simulink model "MyDriveLine_RTW"  (R2022a)
settings: Solver=ode1  StartTime=0.0  StopTime=inf  FixedStep=0.0002  RelTol=1e-3
PreLoadFcn:
  | vehicle = 'Car'; if ~length(which('cmcmd')), cmenv; end
  | MyDriveLine_RTW_bus
InitFcn:
  | vehicle = 'Car'; if ~length(which('cmcmd')), cmenv; end
  | MyDriveLine_RTW_bus
undefined symbols (not defined in the file or in its folder): DiscIntNeverNeededParam
libraries: simulink x3, CarMaker4SL x1
Description:
  | CarMaker Plug-in Model Target
settings Model: ModifiedByFormat=IPG  Creator=IPG  LastModifiedBy=IPG
settings SolverCC: AlgebraicLoopSolver=TrustRegion
settings DataIOCC: LimitDataPoints=on  SaveFormat=Array  SignalLoggingSaveFormat=ModelDataLogs  ReturnWorkspaceOutputs=off
settings OptimizationCC: ExpressionDepthLimit=2147483647  LifeSpan=inf
settings DebuggingCC: UnderspecifiedInitializationDetection=Classic  MergeDetectMultiDrivingBlocksExec=none  FcnCallInpInsideContextMsg=warning  UnconnectedInputMsg=warning  UnconnectedOutputMsg=warning  UnconnectedLineMsg=warning  StateNameClashWarn=warning  SFUnexpectedBacktrackingDiag=warning  SFNoUnconditionalDefaultTransitionDiag=warning  SFMachineParentedDataDiag=warning  ArithmeticOperatorsInVariantConditions=warning
settings HardwareCC: ProdBitPerPointer=32  ProdBitPerSizeT=32  ProdBitPerPtrDiffT=32  ProdLargestAtomicFloat=None  ProdIntDivRoundTo=Undefined  ProdEndianess=Unspecified  ProdWordSize=32  ProdHWDeviceType=32-bit Generic  TargetHWDeviceType=32-bit Generic  ProdEqTarget=off
settings ModelReferenceCC: PropagateSignalLabelsOutOfModel=off
settings SFSimCC: SimUseLocalCustomCode=off  CustomCodeUndefinedFunction=UseInterfaceOnly
settings RTWCC: Description=CarMaker Plug-in Model Target  SystemTargetFile=CarMaker.tlc  TemplateMakefile=CarMaker_unix-win64.tmf  RTWUseLocalCustomCode=off  CustomSourceCode="#include \"SimCore.h\""  DLArmComputeVersion=19.05
settings CodeAppCC: MaxIdLength=63  StateflowObjectComments=on
settings STFCustomTargetCC: ModelReferenceCompliant=off  CodeInterfacePackaging=Reusable function  CPPClassGenCompliant=on  GRTInterface=off  GenerateAllocFcn=on  SystemTargetFile=CarMaker.tlc
settings GRTTargetCC: TargetLangStandard=C89/C90 (ANSI)  ModelReferenceCompliant=off  ParMdlRefBuildCompliant=off  CompOptLevelCompliant=off  ConcurrentExecutionCompliant=off  CombineOutputUpdateFcns=off  MatFileLogging=off  CodeInterfacePackaging=Reusable function  GenerateAllocFcn=on  UseToolchainInfoCompliant=off  ExtModeMexFile=noextcomm
settings ConfigComp: CovMetricSettings=dw  CovSaveCumulativeToWorkspaceVar=on  CovSaveSingleToWorkspaceVar=on  CovExternalEMLEnable=off

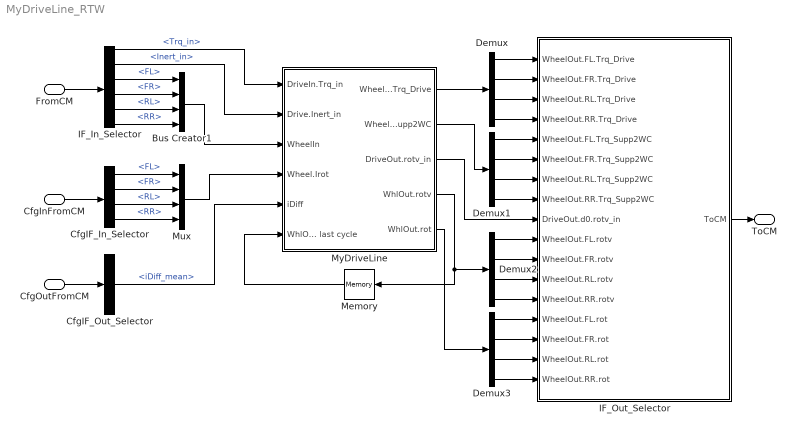
== system MyDriveLine_RTW ==
  FromCM : Inport  OutDataTypeStr=Bus: cmPTDriveLineIn
  CfgInFromCM : Inport  Port=2  OutDataTypeStr=Bus: cmPTDriveLineCfgIn
  CfgOutFromCM : Inport  Port=3  OutDataTypeStr=Bus: cmPTDriveLineCfgOut
  Bus Creator1 : BusCreator  Inputs=4
  CfgIF_In_Selector : BusSelector  OutputSignals=Wheel_Iyy.FL,Wheel_Iyy.FR,Wheel_Iyy.RL,Wheel_Iyy.RR
  CfgIF_Out_Selector : BusSelector  OutputSignals=iDiff_mean
  Demux{,1..3} (4 alike) : Demux
  IF_In_Selector : BusSelector  OutputSignals=DriveIn.d0.Trq_in,DriveIn.d0.Inert_in,WheelIn.FL,WheelIn.FR,WheelIn.RL,WheelIn.RR
  IF_Out_Selector : Subsystem  mask(Signal Selection){}
      mask help: Signal Selection Block
      settings: OpenFcn=cmSignalSelect('SignalSelection_CB',gcb)
  Memory : Memory
  Mux : Mux
  MyDriveLine : Subsystem
  ToCM : Outport  OutDataTypeStr=Bus: cmPTDriveLineOut  VectorParamsAs1DForOutWhenUnconnected=off
  wires:
  FromCM/1 -> IF_In_Selector/1
  IF_Out_Selector/1(ToCM) -> ToCM/1
  CfgInFromCM/1 -> CfgIF_In_Selector/1
  CfgOutFromCM/1 -> CfgIF_Out_Selector/1
  MyDriveLine/1(WheelOut.Trq_Drive) -> Demux/1
  CfgIF_Out_Selector/1 -> MyDriveLine/5(iDiff)  "<iDiff_mean>"
  Demux1/4 -> IF_Out_Selector/8(WheelOut.RR.Trq_Supp2WC)
  MyDriveLine/2(WheelOut.Trq_Supp2WC) -> Demux1/1
  Demux2/1 -> IF_Out_Selector/10(WheelOut.FL.rotv)
  Demux2/2 -> IF_Out_Selector/11(WheelOut.FR.rotv)
  Demux2/3 -> IF_Out_Selector/12(WheelOut.RL.rotv)
  Demux2/4 -> IF_Out_Selector/13(WheelOut.RR.rotv)
  MyDriveLine/4(WhlOut.rotv) -> Demux2/1, Memory/1
  Demux3/1 -> IF_Out_Selector/14(WheelOut.FL.rot)
  Demux3/2 -> IF_Out_Selector/15(WheelOut.FR.rot)
  Demux3/3 -> IF_Out_Selector/16(WheelOut.RL.rot)
  Demux3/4 -> IF_Out_Selector/17(WheelOut.RR.rot)
  MyDriveLine/5(WhlOut.rot) -> Demux3/1
  Memory/1 -> MyDriveLine/6(WhlOut.rotv last cycle)
  Mux/1 -> MyDriveLine/4(Wheel.Irot)
  Bus Creator1/1 -> MyDriveLine/3(WheelIn)
  Demux/1 -> IF_Out_Selector/1(WheelOut.FL.Trq_Drive)
  Demux/2 -> IF_Out_Selector/2(WheelOut.FR.Trq_Drive)
  Demux/3 -> IF_Out_Selector/3(WheelOut.RL.Trq_Drive)
  Demux/4 -> IF_Out_Selector/4(WheelOut.RR.Trq_Drive)
  Demux1/1 -> IF_Out_Selector/5(WheelOut.FL.Trq_Supp2WC)
  Demux1/2 -> IF_Out_Selector/6(WheelOut.FR.Trq_Supp2WC)
  Demux1/3 -> IF_Out_Selector/7(WheelOut.RL.Trq_Supp2WC)
  MyDriveLine/3(DriveOut.rotv_in) -> IF_Out_Selector/9(DriveOut.d0.rotv_in)
  CfgIF_In_Selector/1 -> Mux/1  "<FL>"
  CfgIF_In_Selector/2 -> Mux/2  "<FR>"
  CfgIF_In_Selector/3 -> Mux/3  "<RL>"
  CfgIF_In_Selector/4 -> Mux/4  "<RR>"
  IF_In_Selector/1 -> MyDriveLine/1(DriveIn.Trq_in)  "<Trq_in>"
  IF_In_Selector/2 -> MyDriveLine/2(Drive.Inert_in)  "<Inert_in>"
  IF_In_Selector/3 -> Bus Creator1/1  "<FL>"
  IF_In_Selector/4 -> Bus Creator1/2  "<FR>"
  IF_In_Selector/5 -> Bus Creator1/3  "<RL>"
  IF_In_Selector/6 -> Bus Creator1/4  "<RR>"

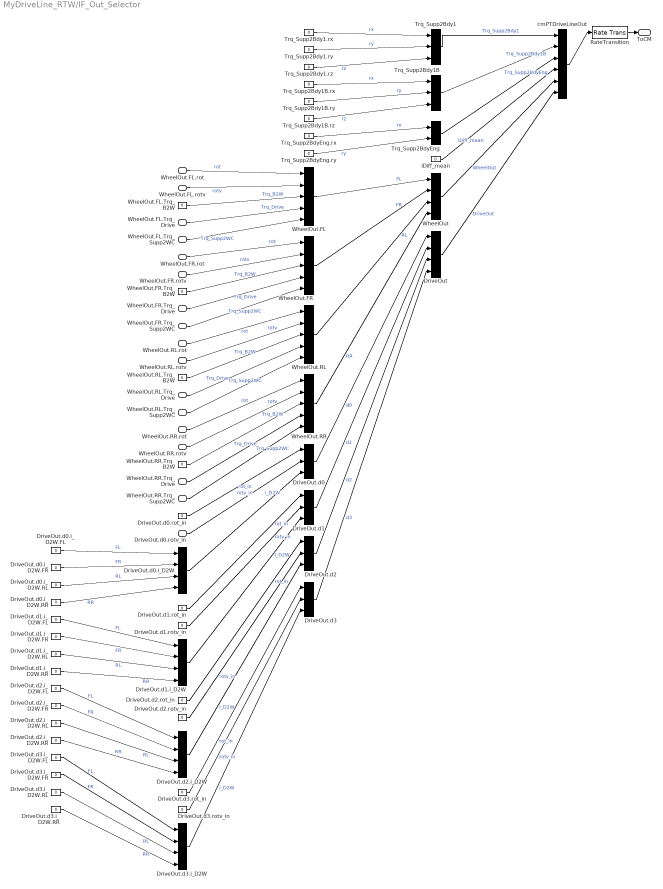
== system MyDriveLine_RTW/IF_Out_Selector ==
  WheelOut.FL.Trq_Drive : Inport
  WheelOut.FR.Trq_Drive : Inport  Port=2
  WheelOut.RL.Trq_Drive : Inport  Port=3
  WheelOut.RR.Trq_Drive : Inport  Port=4
  WheelOut.FL.Trq_Supp2WC : Inport  Port=5
  WheelOut.FR.Trq_Supp2WC : Inport  Port=6
  WheelOut.RL.Trq_Supp2WC : Inport  Port=7
  WheelOut.RR.Trq_Supp2WC : Inport  Port=8
  DriveOut.d0.rotv_in : Inport  Port=9
  WheelOut.FL.rotv : Inport  Port=10
  WheelOut.FR.rotv : Inport  Port=11
  WheelOut.RL.rotv : Inport  Port=12
  WheelOut.RR.rotv : Inport  Port=13
  WheelOut.FL.rot : Inport  Port=14
  WheelOut.FR.rot : Inport  Port=15
  WheelOut.RL.rot : Inport  Port=16
  WheelOut.RR.rot : Inport  Port=17
  DriveOut : BusCreator  Inputs=4
  DriveOut.d{0..3} (4 alike) : BusCreator  Inputs=3
  DriveOut.d0.i_D2W : BusCreator  Inputs=4
  DriveOut.d0.i_D2W.FL : Constant  Value=0
  DriveOut.d0.i_D2W.FR : Constant  Value=0
  DriveOut.d0.i_D2W.RL : Constant  Value=0
  DriveOut.d0.i_D2W.RR : Constant  Value=0
  DriveOut.d0.rot_in : Constant  Value=0
  DriveOut.d1.i_D2W : BusCreator  Inputs=4
  DriveOut.d1.i_D2W.FL : Constant  Value=0
  DriveOut.d1.i_D2W.FR : Constant  Value=0
  DriveOut.d1.i_D2W.RL : Constant  Value=0
  DriveOut.d1.i_D2W.RR : Constant  Value=0
  DriveOut.d1.rot_in : Constant  Value=0
  DriveOut.d1.rotv_in : Constant  Value=0
  DriveOut.d2.i_D2W : BusCreator  Inputs=4
  DriveOut.d2.i_D2W.FL : Constant  Value=0
  DriveOut.d2.i_D2W.FR : Constant  Value=0
  DriveOut.d2.i_D2W.RL : Constant  Value=0
  DriveOut.d2.i_D2W.RR : Constant  Value=0
  DriveOut.d2.rot_in : Constant  Value=0
  DriveOut.d2.rotv_in : Constant  Value=0
  DriveOut.d3.i_D2W : BusCreator  Inputs=4
  DriveOut.d3.i_D2W.FL : Constant  Value=0
  DriveOut.d3.i_D2W.FR : Constant  Value=0
  DriveOut.d3.i_D2W.RL : Constant  Value=0
  DriveOut.d3.i_D2W.RR : Constant  Value=0
  DriveOut.d3.rot_in : Constant  Value=0
  DriveOut.d3.rotv_in : Constant  Value=0
  RateTransition : RateTransition  OutPortSampleTime=str2num(get_param(bdroot,'FixedStep'))
  Trq_Supp2Bdy1 : BusCreator  Inputs=3
  Trq_Supp2Bdy1.rx : Constant  Value=0
  Trq_Supp2Bdy1.ry : Constant  Value=0
  Trq_Supp2Bdy1.rz : Constant  Value=0
  Trq_Supp2Bdy1B : BusCreator  Inputs=3
  Trq_Supp2Bdy1B.rx : Constant  Value=0
  Trq_Supp2Bdy1B.ry : Constant  Value=0
  Trq_Supp2Bdy1B.rz : Constant  Value=0
  Trq_Supp2BdyEng : BusCreator  Inputs=2
  Trq_Supp2BdyEng.rx : Constant  Value=0
  Trq_Supp2BdyEng.ry : Constant  Value=0
  WheelOut : BusCreator  Inputs=4
  WheelOut.FL : BusCreator  Inputs=5
  WheelOut.FL.Trq_B2W : Constant  Value=0
  WheelOut.FR : BusCreator  Inputs=5
  WheelOut.FR.Trq_B2W : Constant  Value=0
  WheelOut.RL : BusCreator  Inputs=5
  WheelOut.RL.Trq_B2W : Constant  Value=0
  WheelOut.RR : BusCreator  Inputs=5
  WheelOut.RR.Trq_B2W : Constant  Value=0
  cmPTDriveLineOut : BusCreator  Inputs=6
  iDiff_mean : Constant  Value=0
  ToCM : Outport  VectorParamsAs1DForOutWhenUnconnected=off
  wires:
  RateTransition/1 -> ToCM/1
  cmPTDriveLineOut/1 -> RateTransition/1
  Trq_Supp2Bdy1/1 -> cmPTDriveLineOut/1  "Trq_Supp2Bdy1"
  Trq_Supp2Bdy1.rx/1 -> Trq_Supp2Bdy1/1  "rx"
  Trq_Supp2Bdy1.ry/1 -> Trq_Supp2Bdy1/2  "ry"
  Trq_Supp2Bdy1.rz/1 -> Trq_Supp2Bdy1/3  "rz"
  Trq_Supp2Bdy1B/1 -> cmPTDriveLineOut/2  "Trq_Supp2Bdy1B"
  Trq_Supp2Bdy1B.rx/1 -> Trq_Supp2Bdy1B/1  "rx"
  Trq_Supp2Bdy1B.ry/1 -> Trq_Supp2Bdy1B/2  "ry"
  Trq_Supp2Bdy1B.rz/1 -> Trq_Supp2Bdy1B/3  "rz"
  Trq_Supp2BdyEng/1 -> cmPTDriveLineOut/3  "Trq_Supp2BdyEng"
  Trq_Supp2BdyEng.rx/1 -> Trq_Supp2BdyEng/1  "rx"
  Trq_Supp2BdyEng.ry/1 -> Trq_Supp2BdyEng/2  "ry"
  iDiff_mean/1 -> cmPTDriveLineOut/4  "iDiff_mean"
  WheelOut/1 -> cmPTDriveLineOut/5  "WheelOut"
  WheelOut.FL/1 -> WheelOut/1  "FL"
  WheelOut.FL.Trq_B2W/1 -> WheelOut.FL/3  "Trq_B2W"
  WheelOut.FR/1 -> WheelOut/2  "FR"
  WheelOut.FR.Trq_B2W/1 -> WheelOut.FR/3  "Trq_B2W"
  WheelOut.RL/1 -> WheelOut/3  "RL"
  WheelOut.RL.Trq_B2W/1 -> WheelOut.RL/3  "Trq_B2W"
  WheelOut.RR/1 -> WheelOut/4  "RR"
  WheelOut.RR.Trq_B2W/1 -> WheelOut.RR/3  "Trq_B2W"
  DriveOut/1 -> cmPTDriveLineOut/6  "DriveOut"
  DriveOut.d0/1 -> DriveOut/1  "d0"
  DriveOut.d0.rot_in/1 -> DriveOut.d0/1  "rot_in"
  DriveOut.d0.i_D2W/1 -> DriveOut.d0/3  "i_D2W"
  DriveOut.d0.i_D2W.FL/1 -> DriveOut.d0.i_D2W/1  "FL"
  DriveOut.d0.i_D2W.FR/1 -> DriveOut.d0.i_D2W/2  "FR"
  DriveOut.d0.i_D2W.RL/1 -> DriveOut.d0.i_D2W/3  "RL"
  DriveOut.d0.i_D2W.RR/1 -> DriveOut.d0.i_D2W/4  "RR"
  DriveOut.d1/1 -> DriveOut/2  "d1"
  DriveOut.d1.rot_in/1 -> DriveOut.d1/1  "rot_in"
  DriveOut.d1.rotv_in/1 -> DriveOut.d1/2  "rotv_in"
  DriveOut.d1.i_D2W/1 -> DriveOut.d1/3  "i_D2W"
  DriveOut.d1.i_D2W.FL/1 -> DriveOut.d1.i_D2W/1  "FL"
  DriveOut.d1.i_D2W.FR/1 -> DriveOut.d1.i_D2W/2  "FR"
  DriveOut.d1.i_D2W.RL/1 -> DriveOut.d1.i_D2W/3  "RL"
  DriveOut.d1.i_D2W.RR/1 -> DriveOut.d1.i_D2W/4  "RR"
  DriveOut.d2/1 -> DriveOut/3  "d2"
  DriveOut.d2.rot_in/1 -> DriveOut.d2/1  "rot_in"
  DriveOut.d2.rotv_in/1 -> DriveOut.d2/2  "rotv_in"
  DriveOut.d2.i_D2W/1 -> DriveOut.d2/3  "i_D2W"
  DriveOut.d2.i_D2W.FL/1 -> DriveOut.d2.i_D2W/1  "FL"
  DriveOut.d2.i_D2W.FR/1 -> DriveOut.d2.i_D2W/2  "FR"
  DriveOut.d2.i_D2W.RL/1 -> DriveOut.d2.i_D2W/3  "RL"
  DriveOut.d2.i_D2W.RR/1 -> DriveOut.d2.i_D2W/4  "RR"
  DriveOut.d3/1 -> DriveOut/4  "d3"
  DriveOut.d3.rot_in/1 -> DriveOut.d3/1  "rot_in"
  DriveOut.d3.rotv_in/1 -> DriveOut.d3/2  "rotv_in"
  DriveOut.d3.i_D2W/1 -> DriveOut.d3/3  "i_D2W"
  DriveOut.d3.i_D2W.FL/1 -> DriveOut.d3.i_D2W/1  "FL"
  DriveOut.d3.i_D2W.FR/1 -> DriveOut.d3.i_D2W/2  "FR"
  DriveOut.d3.i_D2W.RL/1 -> DriveOut.d3.i_D2W/3  "RL"
  DriveOut.d3.i_D2W.RR/1 -> DriveOut.d3.i_D2W/4  "RR"
  WheelOut.FL.Trq_Drive/1 -> WheelOut.FL/4  "Trq_Drive"
  WheelOut.FR.Trq_Drive/1 -> WheelOut.FR/4  "Trq_Drive"
  WheelOut.RL.Trq_Drive/1 -> WheelOut.RL/4  "Trq_Drive"
  WheelOut.RR.Trq_Drive/1 -> WheelOut.RR/4  "Trq_Drive"
  WheelOut.FL.Trq_Supp2WC/1 -> WheelOut.FL/5  "Trq_Supp2WC"
  WheelOut.FR.Trq_Supp2WC/1 -> WheelOut.FR/5  "Trq_Supp2WC"
  WheelOut.RL.Trq_Supp2WC/1 -> WheelOut.RL/5  "Trq_Supp2WC"
  WheelOut.RR.Trq_Supp2WC/1 -> WheelOut.RR/5  "Trq_Supp2WC"
  DriveOut.d0.rotv_in/1 -> DriveOut.d0/2  "rotv_in"
  WheelOut.FL.rotv/1 -> WheelOut.FL/2  "rotv"
  WheelOut.FR.rotv/1 -> WheelOut.FR/2  "rotv"
  WheelOut.RL.rotv/1 -> WheelOut.RL/2  "rotv"
  WheelOut.RR.rotv/1 -> WheelOut.RR/2  "rotv"
  WheelOut.FL.rot/1 -> WheelOut.FL/1  "rot"
  WheelOut.FR.rot/1 -> WheelOut.FR/1  "rot"
  WheelOut.RL.rot/1 -> WheelOut.RL/1  "rot"
  WheelOut.RR.rot/1 -> WheelOut.RR/1  "rot"

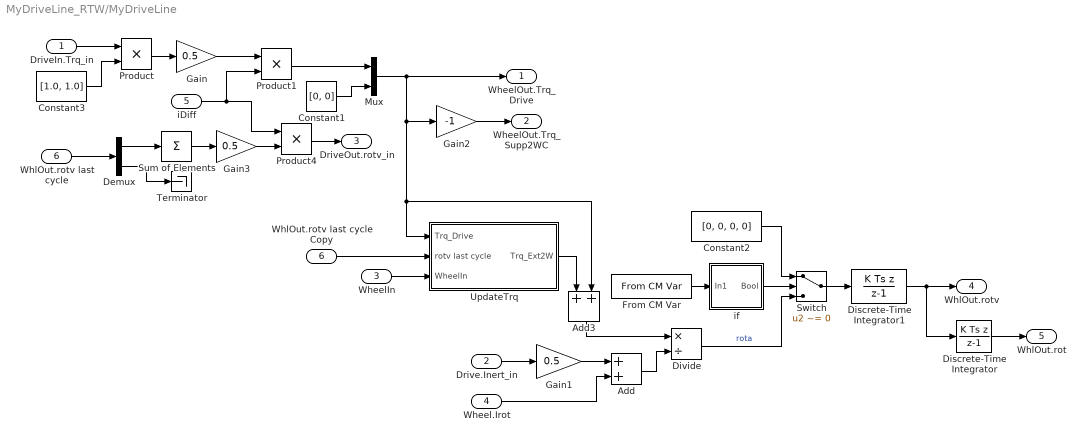
== system MyDriveLine_RTW/MyDriveLine ==
  DriveIn.Trq_in : Inport
  Drive.Inert_in : Inport  Port=2
  WheelIn : Inport  Port=3
  Wheel.Irot : Inport  Port=4
  iDiff : Inport  Port=5
  WhlOut.rotv last cycle : Inport  Port=6
  Add : Sum
  Add3 : Sum
  Constant1 : Constant  Value=[0, 0]
  Constant2 : Constant  Value=[0, 0, 0, 0]
  Constant3 : Constant  Value=[1.0, 1.0]
  Demux : Demux  Outputs=2
  Discrete-Time Integrator : DiscreteIntegrator  IntegratorMethod=Integration: Backward Euler  SampleTime=0.0002  ICPrevOutput=DiscIntNeverNeededParam  ICPrevScaledInput=DiscIntNeverNeededParam
  Discrete-Time Integrator1 : DiscreteIntegrator  IntegratorMethod=Integration: Backward Euler  SampleTime=0.0002  ICPrevOutput=DiscIntNeverNeededParam  ICPrevScaledInput=DiscIntNeverNeededParam
  Divide : Product  Inputs=*/
  From CM Var : CarMaker4SL/From CM Var  xname=SimCore.State
      settings: SourceProductName=CarMaker4SL
  Gain : Gain  Gain=0.5
  Gain1 : Gain  Gain=0.5
  Gain2 : Gain  Gain=-1
  Gain3 : Gain  Gain=0.5
  Mux : Mux  Inputs=2
  Product : Product  RndMeth=Zero
  Product1 : Product  RndMeth=Zero
  Product4 : Product  RndMeth=Zero
  Sum of Elements : Sum  Inputs=+
  Switch : Switch  Criteria=u2 ~= 0  SaturateOnIntegerOverflow=off  InputSameDT=off
  Terminator : Terminator
  UpdateTrq : Subsystem
  WhlOut.rotv last cycle Copy : InportShadow  Port=6
  if : Subsystem
  WheelOut.Trq_Drive : Outport  VectorParamsAs1DForOutWhenUnconnected=off
  WheelOut.Trq_Supp2WC : Outport  Port=2  VectorParamsAs1DForOutWhenUnconnected=off
  DriveOut.rotv_in : Outport  Port=3  VectorParamsAs1DForOutWhenUnconnected=off
  WhlOut.rotv : Outport  Port=4  VectorParamsAs1DForOutWhenUnconnected=off
  WhlOut.rot : Outport  Port=5  VectorParamsAs1DForOutWhenUnconnected=off
  wires:
  Mux/1 -> WheelOut.Trq_Drive/1, UpdateTrq/1(Trq_Drive), Add3/2, Gain2/1
  Constant1/1 -> Mux/2
  Gain/1 -> Product1/1
  Product1/1 -> Mux/1
  iDiff/1 -> Product1/2, Product4/1
  Gain2/1 -> WheelOut.Trq_Supp2WC/1
  Drive.Inert_in/1 -> Gain1/1
  WhlOut.rotv last cycle/1 -> Demux/1
  Demux/1 -> Sum of Elements/1
  Demux/2 -> Terminator/1
  UpdateTrq/1(Trq_Ext2W) -> Add3/1
  WheelIn/1 -> UpdateTrq/3(WheelIn)
  Sum of Elements/1 -> Gain3/1
  Gain3/1 -> Product4/2
  Product4/1 -> DriveOut.rotv_in/1
  Add3/1 -> Divide/1
  Add/1 -> Divide/2
  Switch/1 -> Discrete-Time Integrator1/1
  Divide/1 -> Switch/3  "rota"
  Constant2/1 -> Switch/1
  if/1(Bool) -> Switch/2
  From CM Var/1 -> if/1(In1)
  Discrete-Time Integrator1/1 -> WhlOut.rotv/1, Discrete-Time Integrator/1
  Discrete-Time Integrator/1 -> WhlOut.rot/1
  Gain1/1 -> Add/1
  Product/1 -> Gain/1
  DriveIn.Trq_in/1 -> Product/1
  Constant3/1 -> Product/2
  WhlOut.rotv last cycle Copy/1 -> UpdateTrq/2(rotv last cycle)
  Wheel.Irot/1 -> Add/2

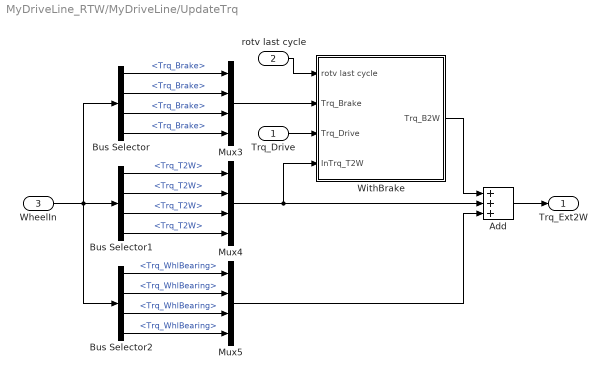
== system MyDriveLine_RTW/MyDriveLine/UpdateTrq ==
  Trq_Drive : Inport
  rotv last cycle : Inport  Port=2
  WheelIn : Inport  Port=3
  Add : Sum  Inputs=+++
  Bus Selector : BusSelector  OutputSignals=FL.Trq_Brake,FR.Trq_Brake,RL.Trq_Brake,RR.Trq_Brake
  Bus Selector1 : BusSelector  OutputSignals=FL.Trq_T2W,FR.Trq_T2W,RL.Trq_T2W,RR.Trq_T2W
  Bus Selector2 : BusSelector  OutputSignals=FL.Trq_WhlBearing,FR.Trq_WhlBearing,RL.Trq_WhlBearing,RR.Trq_WhlBearing
  Mux3 : Mux
  Mux4 : Mux
  Mux5 : Mux
  WithBrake : Subsystem
  Trq_Ext2W : Outport  VectorParamsAs1DForOutWhenUnconnected=off
  wires:
  Mux4/1 -> Add/2, WithBrake/4(InTrq_T2W)
  Mux5/1 -> Add/3
  Trq_Drive/1 -> WithBrake/3(Trq_Drive)
  WithBrake/1(Trq_B2W) -> Add/1
  WheelIn/1 -> Bus Selector/1, Bus Selector1/1, Bus Selector2/1
  Bus Selector/1 -> Mux3/1  "<Trq_Brake>"
  Bus Selector/2 -> Mux3/2  "<Trq_Brake>"
  Bus Selector/3 -> Mux3/3  "<Trq_Brake>"
  Bus Selector/4 -> Mux3/4  "<Trq_Brake>"
  Bus Selector1/1 -> Mux4/1  "<Trq_T2W>"
  Bus Selector1/2 -> Mux4/2  "<Trq_T2W>"
  Bus Selector1/3 -> Mux4/3  "<Trq_T2W>"
  Bus Selector1/4 -> Mux4/4  "<Trq_T2W>"
  Bus Selector2/1 -> Mux5/1  "<Trq_WhlBearing>"
  Bus Selector2/2 -> Mux5/2  "<Trq_WhlBearing>"
  Bus Selector2/3 -> Mux5/3  "<Trq_WhlBearing>"
  Bus Selector2/4 -> Mux5/4  "<Trq_WhlBearing>"
  Add/1 -> Trq_Ext2W/1
  Mux3/1 -> WithBrake/2(Trq_Brake)
  rotv last cycle/1 -> WithBrake/1(rotv last cycle)

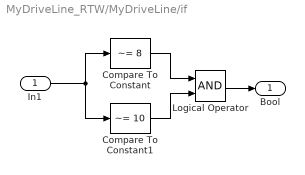
== system MyDriveLine_RTW/MyDriveLine/if ==
  In1 : Inport
  Compare To Constant : simulink/Logic and Bit Operations/Compare To Constant  SystemSampleTime=-1  relop=~=  const=8  LogicOutDataTypeMode=uint8  ZeroCross=off
  Compare To Constant1 : simulink/Logic and Bit Operations/Compare To Constant  SystemSampleTime=-1  relop=~=  const=10  LogicOutDataTypeMode=uint8  ZeroCross=off
  Logical Operator : Logic  AllPortsSameDT=off  OutDataTypeStr=boolean
  Bool : Outport  VectorParamsAs1DForOutWhenUnconnected=off
  wires:
  Logical Operator/1 -> Bool/1
  Compare To Constant/1 -> Logical Operator/1
  Compare To Constant1/1 -> Logical Operator/2
  In1/1 -> Compare To Constant/1, Compare To Constant1/1

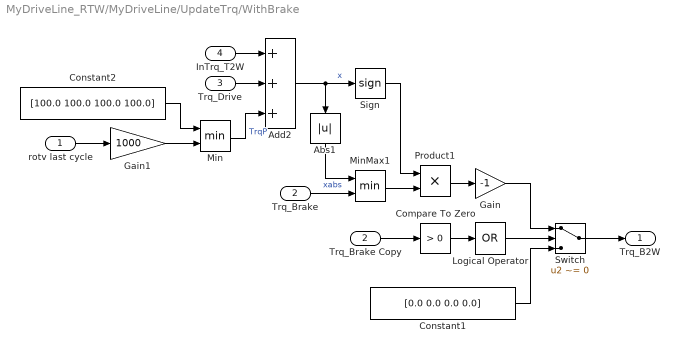
== system MyDriveLine_RTW/MyDriveLine/UpdateTrq/WithBrake ==
  rotv last cycle : Inport
  Trq_Brake : Inport  Port=2
  Trq_Drive : Inport  Port=3
  InTrq_T2W : Inport  Port=4
  Abs1 : Abs  SaturateOnIntegerOverflow=off
  Add2 : Sum  Inputs=+++
  Compare To Zero : simulink/Logic and Bit Operations/Compare To Zero  SystemSampleTime=-1  relop=>  LogicOutDataTypeMode=uint8  ZeroCross=off
  Constant1 : Constant  Value=[0.0 0.0 0.0 0.0]
  Constant2 : Constant  Value=[100.0 100.0 100.0 100.0]
  Gain : Gain  Gain=-1
  Gain1 : Gain  Gain=1000
  Logical Operator : Logic  Operator=OR  Inputs=1  AllPortsSameDT=off  OutDataTypeStr=boolean
  Min : MinMax  Inputs=2
  MinMax1 : MinMax  Inputs=2
  Product1 : Product  RndMeth=Zero
  Sign : Signum
  Switch : Switch  Criteria=u2 ~= 0  SaturateOnIntegerOverflow=off  InputSameDT=off
  Trq_Brake Copy : InportShadow  Port=2
  Trq_B2W : Outport  VectorParamsAs1DForOutWhenUnconnected=off
  wires:
  Add2/1 -> Abs1/1, Sign/1  "x"
  Trq_Brake/1 -> MinMax1/2
  Switch/1 -> Trq_B2W/1
  Product1/1 -> Gain/1
  Compare To Zero/1 -> Logical Operator/1
  Abs1/1 -> MinMax1/1  "xabs"
  Constant1/1 -> Switch/3
  Logical Operator/1 -> Switch/2
  MinMax1/1 -> Product1/2
  Sign/1 -> Product1/1
  Trq_Brake Copy/1 -> Compare To Zero/1
  Constant2/1 -> Min/1
  rotv last cycle/1 -> Gain1/1
  Gain1/1 -> Min/2
  Min/1 -> Add2/3  "TrqP"
  InTrq_T2W/1 -> Add2/1
  Trq_Drive/1 -> Add2/2
  Gain/1 -> Switch/1
